simulink model "hinf_model"  (R2015a)
settings: Solver=ode45  StartTime=0.0  StopTime=10.0  RelTol=1e-3
values from neighbouring files (symbols this model uses):
  Hinf = ss(Hinf_red)    [controller_parameters.m]
  plant = ss(plant)    [controller_parameters.m]
settings Model: CovModelRefEnable=off  Creator=gsavaia  LastModifiedBy=user
settings DataIOCC: SaveFormat=Dataset
settings HardwareCC: ProdBitPerPointer=64  ProdLargestAtomicFloat=Float  ProdIntDivRoundTo=Zero  ProdEndianess=LittleEndian  ProdHWDeviceType=Specified
settings GRTTargetCC: GeneratePreprocessorConditionals=Use local settings

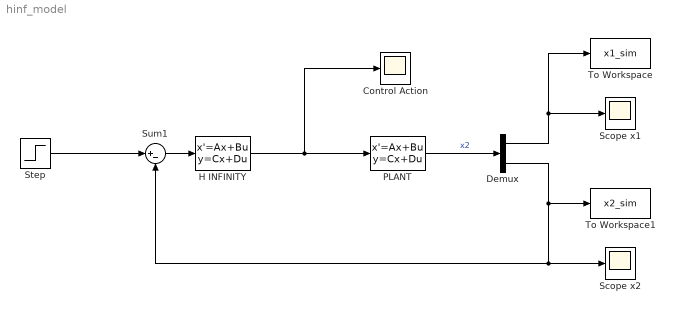
== system hinf_model ==
  Control Action : Scope
      settings: TimeRange=10  YMin=-1  YMax=1  SaveName=ScopeData4
  Demux : Demux  Outputs=2
  H INFINITY : StateSpace  A=Hinf.A  B=Hinf.B  C=Hinf.C  D=Hinf.D  X0=0
  PLANT : StateSpace  A=plant.A  B=plant.B  C=plant.C  D=plant.D  X0=0
  Scope x1 : Scope
      settings: YMin=-0.25393  YMax=2.28535
  Scope x2 : Scope
      settings: YMin=-0.25393  YMax=2.28535
  Step : Step  SampleTime=0
  Sum1 : Sum  Inputs=|+-
  To Workspace : ToWorkspace  VariableName=x1_sim  SampleTime=-1
  To Workspace1 : ToWorkspace  VariableName=x2_sim  SampleTime=-1
  wires:
  Sum1/1 -> H INFINITY/1
  Step/1 -> Sum1/1
  H INFINITY/1 -> PLANT/1, Control Action/1
  PLANT/1 -> Demux/1  "x2"
  Demux/1 -> To Workspace/1, Scope x1/1
  Demux/2 -> Scope x2/1, Sum1/2, To Workspace1/1
